simulink model "BoatBoat"  (R2020a)
settings: Solver=VariableStepAuto  StartTime=0.0  StopTime=5  RelTol=1e-3
libraries: fuzblock x1
settings Model: Creator=Donald  LastModifiedBy=Donald

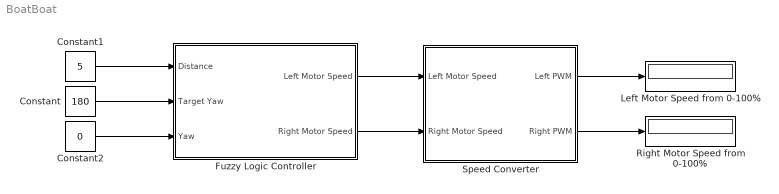
== system BoatBoat ==
  Constant : Constant  Value=180
  Constant1 : Constant  Value=5
  Constant2 : Constant  Value=0
  Fuzzy Logic Controller : Subsystem
  Left Motor Speed from 0-100% : Display
  Right Motor Speed from 0-100% : Display
  Speed Converter : Subsystem
  wires:
  Fuzzy Logic Controller/1(Left Motor Speed) -> Speed Converter/1(Left Motor Speed)
  Speed Converter/1(Left PWM) -> Left Motor Speed from 0-100%/1
  Speed Converter/2(Right PWM) -> Right Motor Speed from 0-100%/1
  Fuzzy Logic Controller/2(Right Motor Speed) -> Speed Converter/2(Right Motor Speed)
  Constant2/1 -> Fuzzy Logic Controller/3(Yaw)
  Constant/1 -> Fuzzy Logic Controller/2(Target Yaw)
  Constant1/1 -> Fuzzy Logic Controller/1(Distance)

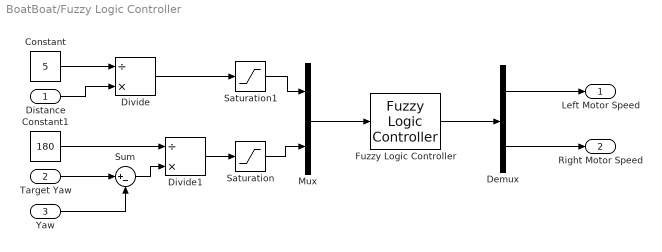
== system BoatBoat/Fuzzy Logic Controller ==
  Distance : Inport
  Target Yaw : Inport  Port=2
  Yaw : Inport  Port=3
  Constant : Constant  Value=5
  Constant1 : Constant  Value=180
  Demux : Demux  Outputs=2
  Divide : Product  Inputs=/*
  Divide1 : Product  Inputs=/*
  Fuzzy Logic Controller : fuzblock/Fuzzy Logic  Controller  FIS='Motor_Mixing_Algorithm.fis'  OutputSampleNumber=101  DataType=double  FuzzifiedInputs=off  RuleFiringStrengths=off  RuleOutputs=off  AggregatedOutputs=off  SimulateUsing=Interpreted execution  OutOfRangeInputValueMessage=warning  NoRuleFiredMessage=warning  EmptyOutputFuzzySetMessage=warning
  Mux : Mux  Inputs=2
  Saturation : Saturate  UpperLimit=1  LowerLimit=-1
  Saturation1 : Saturate  UpperLimit=1  LowerLimit=0
  Sum : Sum  Inputs=|+-
  Left Motor Speed : Outport
  Right Motor Speed : Outport  Port=2
  wires:
  Mux/1 -> Fuzzy Logic Controller/1
  Target Yaw/1 -> Sum/1
  Yaw/1 -> Sum/2
  Saturation/1 -> Mux/2
  Saturation1/1 -> Mux/1
  Distance/1 -> Divide/2
  Divide/1 -> Saturation1/1
  Constant/1 -> Divide/1
  Divide1/1 -> Saturation/1
  Constant1/1 -> Divide1/1
  Sum/1 -> Divide1/2
  Demux/1 -> Left Motor Speed/1
  Demux/2 -> Right Motor Speed/1
  Fuzzy Logic Controller/1 -> Demux/1

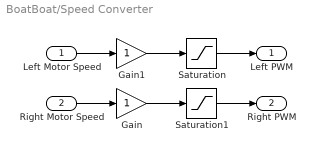
== system BoatBoat/Speed Converter ==
  Left Motor Speed : Inport
  Right Motor Speed : Inport  Port=2
  Gain : Gain
  Gain1 : Gain
  Saturation : Saturate  UpperLimit=100  LowerLimit=0
  Saturation1 : Saturate  UpperLimit=100  LowerLimit=0
  Left PWM : Outport
  Right PWM : Outport  Port=2
  wires:
  Right Motor Speed/1 -> Gain/1
  Left Motor Speed/1 -> Gain1/1
  Gain/1 -> Saturation1/1
  Gain1/1 -> Saturation/1
  Saturation/1 -> Left PWM/1
  Saturation1/1 -> Right PWM/1
